simulink model "rigidBodyControl"  (R2016b)
settings: Solver=VariableStepAuto  StartTime=0.0  StopTime=0.3  FixedStep=2e-4  RelTol=1e-3
values from neighbouring files (symbols this model uses):
  denGc = denGc{1}    [rigidBodyInit.m]
  denGp = [m0 0 0]    [rigidBodyInit.m]
  fs = 5000    [rigidBodyInit.m]
  numGc = numGc{1}    [rigidBodyInit.m]
  numGp = [1]    [rigidBodyInit.m]
  Ts = 1/fs    (= 0.0002)    [rigidBodyInit.m]
libraries: simulink x3, model_controller x1
settings Model: Creator=Dai Luyao  LastModifiedBy=Dai Luyao

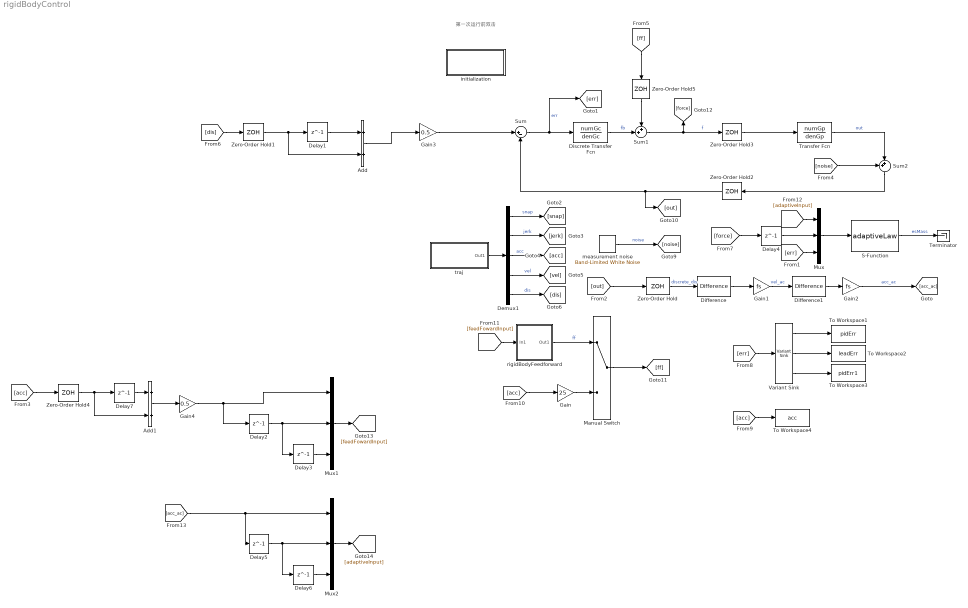
== system rigidBodyControl ==
  note: 第一次运行前双击
  Add : Sum
  Add1 : Sum
  Delay{1..7} (7 alike) : Delay  DelayLength=1
  Demux1 : Demux  Outputs=5
  Difference : simulink/Discrete/Difference  ICPrevInput=0.0  OutMin=[]  OutMax=[]  OutDataType=fixdt(1, 16)  OutScaling=2^-10  DoSatur=off
  Difference1 : simulink/Discrete/Difference  ICPrevInput=0.0  OutMin=[]  OutMax=[]  OutDataType=fixdt(1, 16)  OutScaling=2^-10  DoSatur=off
  Discrete Transfer Fcn : DiscreteTransferFcn  Numerator=numGc  Denominator=denGc  SampleTime=Ts
  Gain : Gain  Gain=25
  Gain1 : Gain  Gain=fs
  Gain2 : Gain  Gain=fs
  Gain3 : Gain  Gain=0.5
  Gain4 : Gain  Gain=0.5
  Manual Switch : ManualSwitch
  Mux : Mux  Inputs=3
  Mux1 : Mux  Inputs=3
  Mux2 : Mux  Inputs=3
  S-Function : S-Function  FunctionName=adaptiveLaw  Parameters=1  SFunctionDeploymentMode=off  EnableBusSupport=off
  Sum : Sum  Inputs=|+-
  Sum1 : Sum  Inputs=++|
  Sum2 : Sum  Inputs=++|
  Terminator : Terminator
  To Workspace1 : ToWorkspace  VariableName=pidErr  SaveFormat=Structure With Time  SampleTime=-1
  To Workspace2 : ToWorkspace  VariableName=leadErr  SaveFormat=Structure With Time  SampleTime=-1
  To Workspace3 : ToWorkspace  VariableName=pidErr1  SaveFormat=Structure With Time  SampleTime=-1
  To Workspace4 : ToWorkspace  VariableName=acc  SaveFormat=Structure With Time  SampleTime=-1
  Transfer Fcn : TransferFcn  Numerator=numGp  Denominator=denGp
  Variant Sink : VariantSink
  Zero-Order Hold{,1..5} (6 alike) : ZeroOrderHold  SampleTime=Ts
  initialization : Subsystem
      settings: OpenFcn=rigidBodyInit;  MoveFcn=edit rigidBodyInit;
  measurement noise : simulink/Sources/Band-Limited White Noise  Cov=noisePower  Ts=Ts  seed=[23341]
  rigidBodyFeedforward : Subsystem
  traj : Subsystem  BlockChoice=4th order traj
      link override 3rd order traj: j=800  v=0.25  x=0.06  a=10
      settings: AttributesFormatString=%<BlockChoice>  TemplateBlock=model_controller/Profile Generators/traj  MemberBlocks=2th order traj,3rd order traj,4th order traj,step
  wires:
  Sum/1 -> Discrete Transfer Fcn/1, [err]  "err"
  Discrete Transfer Fcn/1 -> Sum1/2  "fb"
  Sum1/1 -> Zero-Order Hold3/1, [force]  "f"
  Difference1/1 -> Gain2/1
  Difference/1 -> Gain1/1
  Gain1/1 -> Difference1/1  "vel_ac"
  Mux/1 -> S-Function/1
  S-Function/1 -> Terminator/1  "esMass"
  [adaptiveInput] -> Mux/1
  Zero-Order Hold/1 -> Difference/1  "discrete_dis"
  [err] -> Mux/3
  measurement noise/1 -> [noise]  "noise"
  Transfer Fcn/1 -> Sum2/2  "out"
  [noise] -> Sum2/1
  Demux1/1 -> [snap]  "snap"
  Demux1/2 -> [jerk]  "jerk"
  Demux1/3 -> [acc]  "acc"
  Demux1/4 -> [vel]  "vel"
  Demux1/5 -> [dis]  "dis"
  traj/1(Out1) -> Demux1/1
  [out] -> Zero-Order Hold/1
  rigidBodyFeedforward/1(Out1) -> Manual Switch/1  "ff"
  [err] -> Variant Sink/1
  Variant Sink/1 -> To Workspace1/1
  Variant Sink/2 -> To Workspace2/1
  Variant Sink/3 -> To Workspace3/1
  [acc] -> To Workspace4/1
  Manual Switch/1 -> [ff]
  [acc] -> Gain/1
  Gain/1 -> Manual Switch/2
  Gain2/1 -> [acc_ac]  "acc_ac"
  Delay3/1 -> Mux1/3
  Delay2/1 -> Delay3/1, Mux1/2
  Mux1/1 -> [feedFowardInput]
  [feedFowardInput] -> rigidBodyFeedforward/1(In1)
  Delay6/1 -> Mux2/3
  Delay5/1 -> Mux2/2, Delay6/1
  [acc_ac] -> Mux2/1, Delay5/1
  Mux2/1 -> [adaptiveInput]
  Gain3/1 -> Sum/1
  Delay1/1 -> Add/1
  Add/1 -> Gain3/1
  [dis] -> Zero-Order Hold1/1
  Zero-Order Hold1/1 -> Add/2, Delay1/1
  Sum2/1 -> Zero-Order Hold2/1
  Zero-Order Hold2/1 -> [out], Sum/2
  [force] -> Delay4/1
  Delay4/1 -> Mux/2
  Zero-Order Hold3/1 -> Transfer Fcn/1
  [acc] -> Zero-Order Hold4/1
  [ff] -> Zero-Order Hold5/1
  Zero-Order Hold5/1 -> Sum1/1
  Zero-Order Hold4/1 -> Add1/2, Delay7/1
  Delay7/1 -> Add1/1
  Add1/1 -> Gain4/1
  Gain4/1 -> Delay2/1, Mux1/1

== system rigidBodyControl/initialization ==

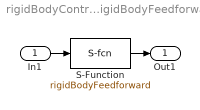
== system rigidBodyControl/rigidBodyFeedforward ==
  In1 : Inport
  S-Function : S-Function  FunctionName=rigidBodyFeedforward  SFunctionDeploymentMode=off  EnableBusSupport=off
  Out1 : Outport
  wires:
  In1/1 -> S-Function/1
  S-Function/1 -> Out1/1

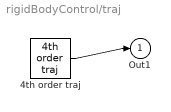
== system rigidBodyControl/traj ==
  4th order traj : model_controller/Profile Generators/4th order traj  t0=0  x=0.06  v=0.25  a=10  j=800  d=64000  Ts=0
  Out1 : Outport
  wires:
  4th order traj/1 -> Out1/1
